simulink model "RWA_Controller"  (R2017a)
settings: Solver=VariableStepAuto  StartTime=0  StopTime=ts+60  FixedStep=0.01  RelTol=1e-3
InitFcn:
  | Init_Sim
values from neighbouring files (symbols this model uses):
  I = [0.07920140 0.00973142 0.00215335 ... (first row only)    [Init_Sim.m]
  J = Jw + Jm    (= 2.539e-05)    [Init_Sim.m]
  K = [k1  0   0   0 ... (first row only)    [Init_Sim.m]    (also in animate.m = eciunitvecs(:,3))
  Kd = 2*zeta*wn    (= 0.133333333333)    [Init_Sim.m]
  Ke = 1/(56*pi)    (= 0.00568410511042)    [Init_Sim.m]
  Kp = 2*wn^2    (= 0.00888888888889)    [Init_Sim.m]
  Kt = 5.67e-3    (= 0.00567)    [Init_Sim.m]
  phi_d = 0    [Init_Sim.m]
  phi_d0 = 0    [Init_Sim.m]
  psi_d = -90    [Init_Sim.m]
  psi_d0 = 0    [Init_Sim.m]
  r = [0.00004275; -0.00008398; -0.9099]*10^(-3)    [Init_Sim.m]    (also in csacs_nonlinear_dyn.m = [r_temp(1) r_temp(2) r_temp(3)]')
  T = [ cos(beta)            0        sin(beta) ... (first row only)    [Init_Sim.m]
  theta_d = 0    [Init_Sim.m]
  theta_d0 = 0    [Init_Sim.m]
  W = [w1   0   0   0 ... (first row only)    [Init_Sim.m]
  wn = 4/(zeta*ts)    (= 0.0666666666667)    [Init_Sim.m]
  x0 = [q_0(1); q_0(2); q_0(3); q_0(4); wb_0(1); wb_0(2); wb_0(3)]    [Init_Sim.m]
  zeta = 1    [Init_Sim.m]
settings Model: Creator=Anthony  LastModifiedBy=Anthony

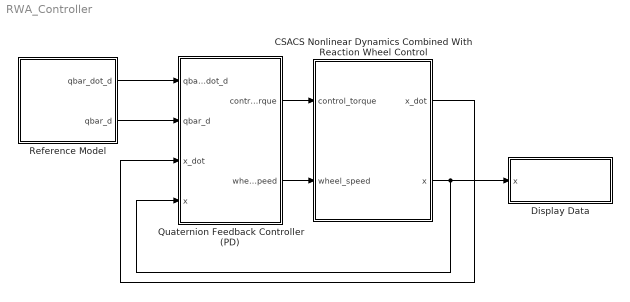
== system RWA_Controller ==
  CSACS Nonlinear Dynamics Combined With Reaction Wheel Control : Subsystem
  Display Data : Subsystem
  Quaternion Feedback Controller (PD) : Subsystem
  Reference Model : Subsystem
  wires:
  Reference Model/1(qbar_dot_d) -> Quaternion Feedback Controller (PD)/1(qbar_dot_d)
  Reference Model/2(qbar_d) -> Quaternion Feedback Controller (PD)/2(qbar_d)
  Quaternion Feedback Controller (PD)/1(control_torque) -> CSACS Nonlinear Dynamics Combined With Reaction Wheel Control/1("control_torque ")
  CSACS Nonlinear Dynamics Combined With Reaction Wheel Control/1(x_dot) -> Quaternion Feedback Controller (PD)/3(x_dot)
  CSACS Nonlinear Dynamics Combined With Reaction Wheel Control/2(x) -> Display Data/1(x), Quaternion Feedback Controller (PD)/4(x)
  Quaternion Feedback Controller (PD)/2(wheel_speed) -> CSACS Nonlinear Dynamics Combined With Reaction Wheel Control/2(wheel_speed)

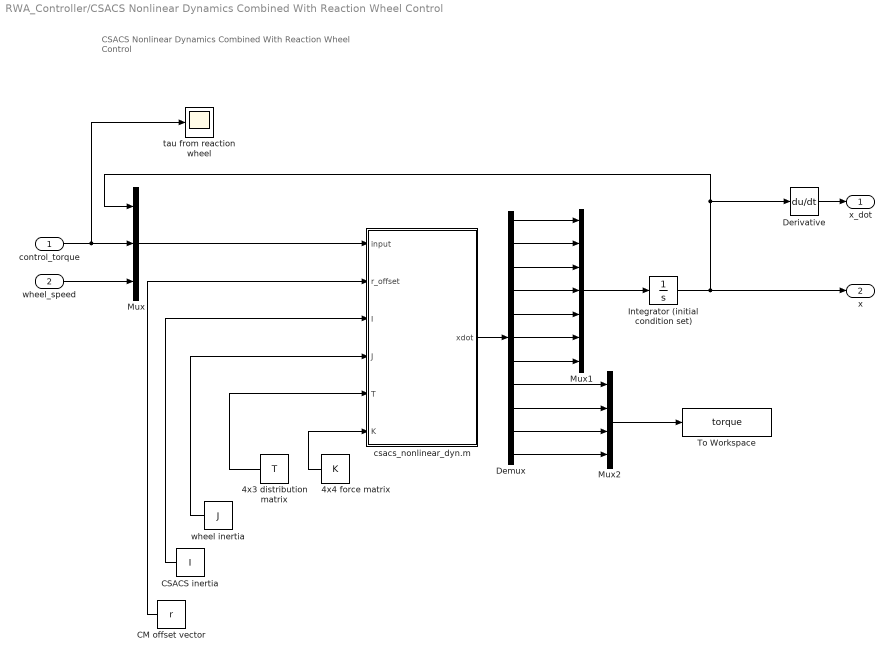
== system RWA_Controller/CSACS Nonlinear Dynamics Combined With Reaction Wheel Control ==
  note: CSACS Nonlinear Dynamics Combined
      | With Reaction Wheel Control
  "control_torque " : Inport
  wheel_speed : Inport  Port=2
  4x3 distribution matrix : Constant  Value=T  VectorParams1D=off
  4x4 force matrix : Constant  Value=K  VectorParams1D=off
  CM offset vector : Constant  Value=r  VectorParams1D=off
  CSACS inertia : Constant  Value=I  VectorParams1D=off
  Demux : Demux  Outputs=11
  Derivative : Derivative
  Integrator (initial condition set) : Integrator  InitialCondition=x0
  Mux : Mux  Inputs=3
  Mux1 : Mux  Inputs=7
  Mux2 : Mux
  To Workspace : ToWorkspace  VariableName=torque  SaveFormat=Timeseries  SampleTime=-1
  csacs_nonlinear_dyn.m : MATLAB Function  TreatAsAtomicUnit=on
  tau from reaction wheel : Scope
  wheel inertia : Constant  Value=J  VectorParams1D=off
  x_dot : Outport
  x : Outport  Port=2
  wires:
  Mux/1 -> csacs_nonlinear_dyn.m/1(input)
  "control_torque "/1 -> Mux/2, tau from reaction wheel/1
  csacs_nonlinear_dyn.m/1(xdot) -> Demux/1
  Demux/1 -> Mux1/1
  Demux/2 -> Mux1/2
  Demux/3 -> Mux1/3
  Demux/4 -> Mux1/4
  Demux/5 -> Mux1/5
  Demux/6 -> Mux1/6
  Demux/7 -> Mux1/7
  Demux/8 -> Mux2/1
  Demux/9 -> Mux2/2
  Demux/10 -> Mux2/3
  Demux/11 -> Mux2/4
  Mux1/1 -> Integrator (initial condition set)/1
  Derivative/1 -> x_dot/1
  Integrator (initial condition set)/1 -> x/1, Derivative/1, Mux/1
  Mux2/1 -> To Workspace/1
  4x4 force matrix/1 -> csacs_nonlinear_dyn.m/6(K)
  4x3 distribution matrix/1 -> csacs_nonlinear_dyn.m/5(T)
  CSACS inertia/1 -> csacs_nonlinear_dyn.m/3(I)
  CM offset vector/1 -> csacs_nonlinear_dyn.m/2(r_offset)
  wheel_speed/1 -> Mux/3
  wheel inertia/1 -> csacs_nonlinear_dyn.m/4(J)

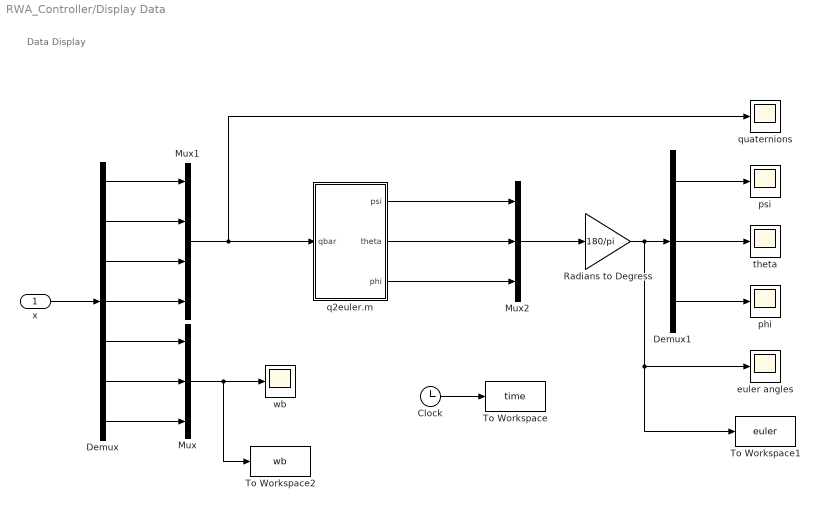
== system RWA_Controller/Display Data ==
  note: Data Display
  x : Inport
  Clock : Clock
      settings: Decimation=100
  Demux : Demux  Outputs=7
  Demux1 : Demux  Outputs=3
  Mux : Mux  Inputs=3
  Mux1 : Mux
  Mux2 : Mux  Inputs=3
  Radians to Degress : Gain  Gain=180/pi
  To Workspace : ToWorkspace  VariableName=time  SaveFormat=Timeseries  SampleTime=-1
  To Workspace1 : ToWorkspace  VariableName=euler  SaveFormat=Timeseries  SampleTime=-1
  To Workspace2 : ToWorkspace  VariableName=wb  SaveFormat=Timeseries  SampleTime=-1
  euler angles : Scope
  phi : Scope
  psi : Scope
  q2euler.m : MATLAB Function  TreatAsAtomicUnit=on
  quaternions : Scope
  theta : Scope
  wb : Scope
  wires:
  x/1 -> Demux/1
  Demux/1 -> Mux1/1
  Demux/2 -> Mux1/2
  Demux/3 -> Mux1/3
  Demux/4 -> Mux1/4
  Demux/6 -> Mux/2
  Demux/5 -> Mux/1
  Demux/7 -> Mux/3
  Demux1/1 -> psi/1
  Demux1/2 -> theta/1
  Demux1/3 -> phi/1
  Mux2/1 -> Radians to Degress/1
  Mux1/1 -> quaternions/1, q2euler.m/1(qbar)
  Clock/1 -> To Workspace/1
  Radians to Degress/1 -> euler angles/1, To Workspace1/1, Demux1/1
  Mux/1 -> To Workspace2/1, wb/1
  q2euler.m/1(psi) -> Mux2/1
  q2euler.m/2(theta) -> Mux2/2
  q2euler.m/3(phi) -> Mux2/3

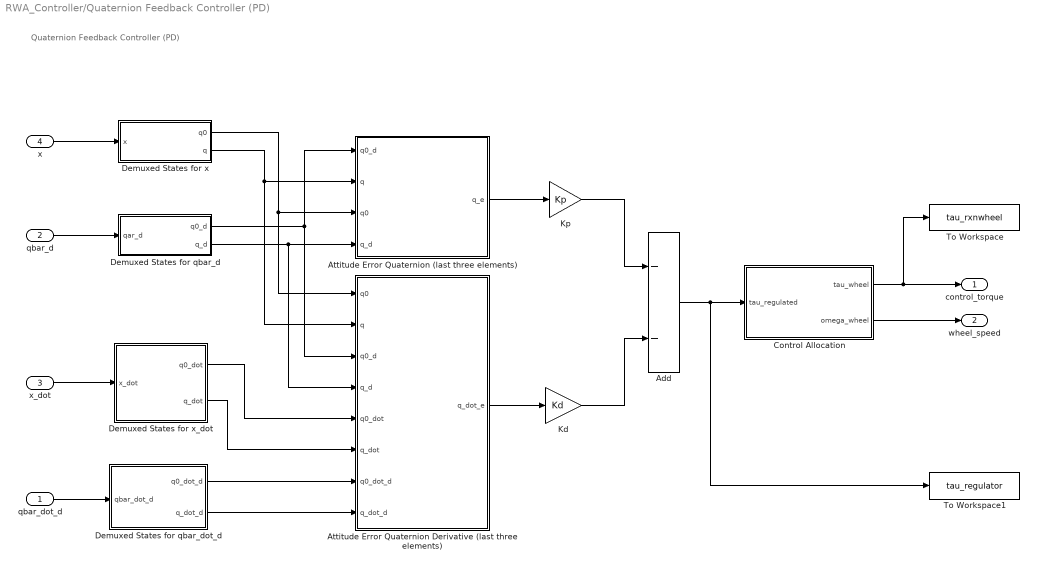
== system RWA_Controller/Quaternion Feedback Controller (PD) ==
  note: Quaternion Feedback Controller (PD)
  qbar_dot_d : Inport
  qbar_d : Inport  Port=2
  x_dot : Inport  Port=3
  x : Inport  Port=4
  Add : Sum  Inputs=--
  Attitude Error Quaternion (last three elements) : Subsystem
  Attitude Error Quaternion Derivative (last three elements) : Subsystem
  Control Allocation : Subsystem
  Demuxed States for qbar_d : Subsystem
  Demuxed States for qbar_dot_d : Subsystem
  Demuxed States for x : Subsystem
  Demuxed States for x_dot : Subsystem
  Kd : Gain  Gain=Kd
  Kp : Gain  Gain=Kp
  To Workspace : ToWorkspace  VariableName=tau_rxnwheel  SaveFormat=Timeseries  SampleTime=-1
  To Workspace1 : ToWorkspace  VariableName=tau_regulator  SaveFormat=Timeseries  SampleTime=-1
  control_torque : Outport
  wheel_speed : Outport  Port=2
  wires:
  qbar_dot_d/1 -> Demuxed States for qbar_dot_d/1(qbar_dot_d)
  qbar_d/1 -> Demuxed States for qbar_d/1(qar_d)
  x_dot/1 -> Demuxed States for x_dot/1(x_dot)
  x/1 -> Demuxed States for x/1(x)
  Demuxed States for x/1(q0) -> Attitude Error Quaternion Derivative (last three elements)/1(q0), Attitude Error Quaternion (last three elements)/3(q0)
  Demuxed States for x/2(q) -> Attitude Error Quaternion Derivative (last three elements)/2(q), Attitude Error Quaternion (last three elements)/2(q)
  Demuxed States for qbar_d/1(q0_d) -> Attitude Error Quaternion Derivative (last three elements)/3(q0_d), Attitude Error Quaternion (last three elements)/1(q0_d)
  Demuxed States for qbar_d/2(q_d) -> Attitude Error Quaternion Derivative (last three elements)/4(q_d), Attitude Error Quaternion (last three elements)/4(q_d)
  Demuxed States for qbar_dot_d/2(q_dot_d) -> Attitude Error Quaternion Derivative (last three elements)/8(q_dot_d)
  Demuxed States for qbar_dot_d/1(q0_dot_d) -> Attitude Error Quaternion Derivative (last three elements)/7(q0_dot_d)
  Demuxed States for x_dot/1(q0_dot) -> Attitude Error Quaternion Derivative (last three elements)/5(q0_dot)
  Demuxed States for x_dot/2(q_dot) -> Attitude Error Quaternion Derivative (last three elements)/6(q_dot)
  Attitude Error Quaternion Derivative (last three elements)/1(q_dot_e) -> Kd/1
  Attitude Error Quaternion (last three elements)/1(q_e) -> Kp/1
  Kp/1 -> Add/1
  Kd/1 -> Add/2
  Control Allocation/1(tau_wheel) -> control_torque/1, To Workspace/1
  Add/1 -> To Workspace1/1, Control Allocation/1(tau_regulated)
  Control Allocation/2(omega_wheel) -> wheel_speed/1

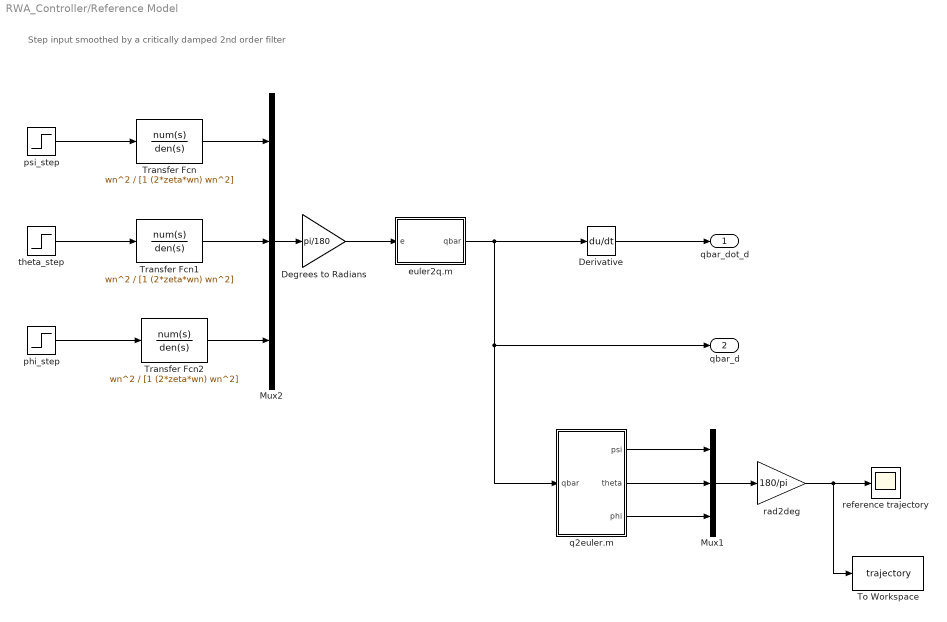
== system RWA_Controller/Reference Model ==
  note: Step input smoothed by a critically damped 2nd order filter
  Degrees to Radians : Gain  Gain=pi/180
  Derivative : Derivative
  Mux1 : Mux  Inputs=3
  Mux2 : Mux  Inputs=3
  To Workspace : ToWorkspace  VariableName=trajectory  SaveFormat=Timeseries  SampleTime=-1
  Transfer Fcn : TransferFcn  Numerator=wn^2  Denominator=[1 (2*zeta*wn) wn^2]
  Transfer Fcn1 : TransferFcn  Numerator=wn^2  Denominator=[1 (2*zeta*wn) wn^2]
  Transfer Fcn2 : TransferFcn  Numerator=wn^2  Denominator=[1 (2*zeta*wn) wn^2]
  euler2q.m : MATLAB Function  TreatAsAtomicUnit=on
  phi_step : Step  Before=phi_d0  After=phi_d  SampleTime=0
  "psi_step " : Step  Before=psi_d0  After=psi_d  SampleTime=0
  q2euler.m : MATLAB Function  TreatAsAtomicUnit=on
  rad2deg : Gain  Gain=180/pi
  reference trajectory : Scope
  theta_step : Step  Before=theta_d0  After=theta_d  SampleTime=0
  qbar_dot_d : Outport
  qbar_d : Outport  Port=2
  wires:
  theta_step/1 -> Transfer Fcn1/1
  Transfer Fcn2/1 -> Mux2/3
  Transfer Fcn1/1 -> Mux2/2
  phi_step/1 -> Transfer Fcn2/1
  "psi_step "/1 -> Transfer Fcn/1
  euler2q.m/1(qbar) -> qbar_d/1, q2euler.m/1(qbar), Derivative/1
  q2euler.m/2(theta) -> Mux1/2
  Degrees to Radians/1 -> euler2q.m/1(e)
  rad2deg/1 -> To Workspace/1, reference trajectory/1
  q2euler.m/1(psi) -> Mux1/1
  q2euler.m/3(phi) -> Mux1/3
  Derivative/1 -> qbar_dot_d/1
  Mux1/1 -> rad2deg/1
  Mux2/1 -> Degrees to Radians/1
  Transfer Fcn/1 -> Mux2/1

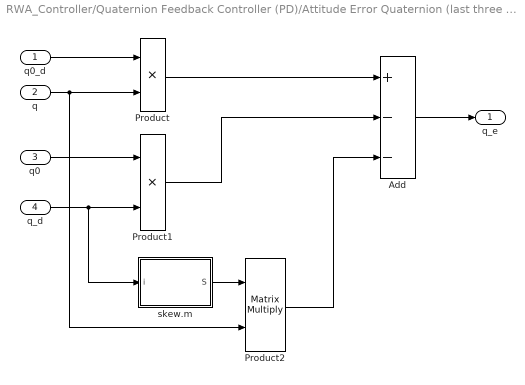
== system RWA_Controller/Quaternion Feedback Controller (PD)/Attitude Error Quaternion (last three elements) ==
  q0_d : Inport
  q : Inport  Port=2
  q0 : Inport  Port=3
  q_d : Inport  Port=4
  Add : Sum  Inputs=+--
  Product : Product
  Product1 : Product
  Product2 : Product  Multiplication=Matrix(*)
  skew.m : MATLAB Function  TreatAsAtomicUnit=on
  q_e : Outport
  wires:
  skew.m/1(S) -> Product2/1
  q0_d/1 -> Product/1
  q0/1 -> Product1/1
  q_d/1 -> skew.m/1(i), Product1/2
  q/1 -> Product2/2, Product/2
  Product/1 -> Add/1
  Product1/1 -> Add/2
  Add/1 -> q_e/1
  Product2/1 -> Add/3

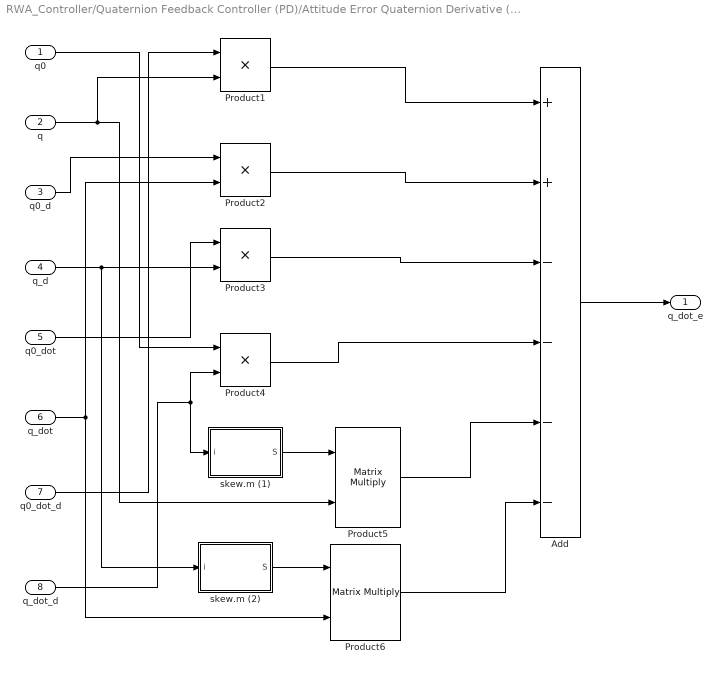
== system RWA_Controller/Quaternion Feedback Controller (PD)/Attitude Error Quaternion Derivative (last three elements) ==
  q0 : Inport
  q : Inport  Port=2
  q0_d : Inport  Port=3
  q_d : Inport  Port=4
  q0_dot : Inport  Port=5
  q_dot : Inport  Port=6
  q0_dot_d : Inport  Port=7
  q_dot_d : Inport  Port=8
  Add : Sum  Inputs=++----
  Product{1..4} (4 alike) : Product
  Product5 : Product  Multiplication=Matrix(*)
  Product6 : Product  Multiplication=Matrix(*)
  skew.m (1) : MATLAB Function  TreatAsAtomicUnit=on
  skew.m (2) : MATLAB Function  TreatAsAtomicUnit=on
  q_dot_e : Outport
  wires:
  Add/1 -> q_dot_e/1
  q0/1 -> Product4/1
  q_dot_d/1 -> skew.m (1)/1(i), Product4/2
  q_d/1 -> skew.m (2)/1(i), Product3/2
  q0_dot/1 -> Product3/1
  q0_dot_d/1 -> Product1/1
  skew.m (2)/1(S) -> Product6/1
  q_dot/1 -> Product6/2, Product2/2
  skew.m (1)/1(S) -> Product5/1
  q/1 -> Product5/2, Product1/2
  q0_d/1 -> Product2/1
  Product1/1 -> Add/1
  Product2/1 -> Add/2
  Product3/1 -> Add/3
  Product4/1 -> Add/4
  Product5/1 -> Add/5
  Product6/1 -> Add/6

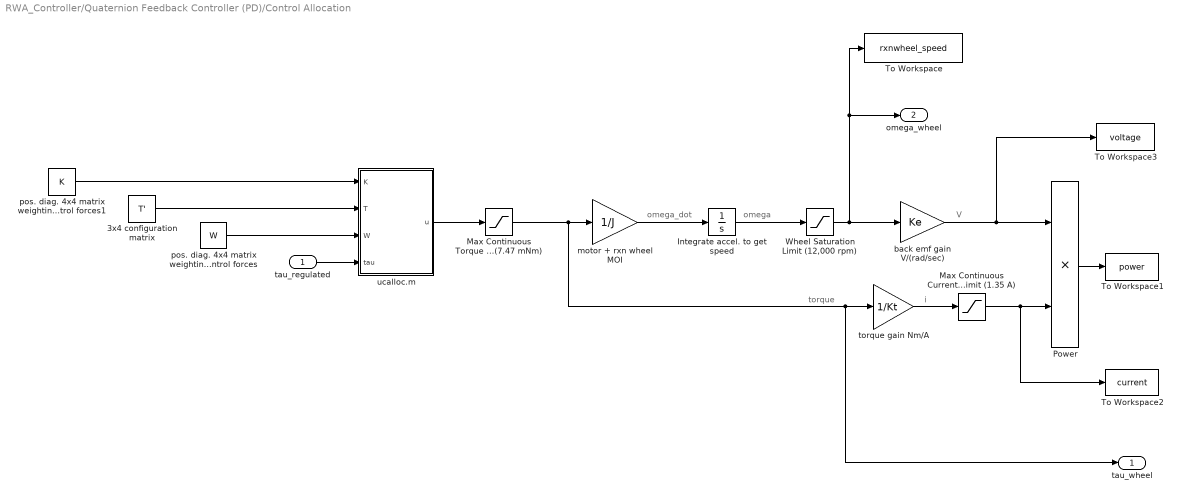
== system RWA_Controller/Quaternion Feedback Controller (PD)/Control Allocation ==
  note: torque
  note: omega
  note: omega_dot
  note: i
  note: V
  tau_regulated : Inport
  3x4 configuration matrix : Constant  Value=T'  VectorParams1D=off
  Integrate accel. to get speed : Integrator
  Max Continuous Current Limit (1.35 A) : Saturate  UpperLimit=12e3*(pi/30)  LowerLimit=-12e3*(pi/30)
  Max Continuous Torque Limit (7.47 mNm) : Saturate  UpperLimit=7.47e-3  LowerLimit=-7.47e-3
  Power : Product
  To Workspace : ToWorkspace  VariableName=rxnwheel_speed  SaveFormat=Timeseries  SampleTime=-1
  To Workspace1 : ToWorkspace  VariableName=power  SaveFormat=Timeseries  SampleTime=-1
  To Workspace2 : ToWorkspace  VariableName=current  SaveFormat=Timeseries  SampleTime=-1
  To Workspace3 : ToWorkspace  VariableName=voltage  SaveFormat=Timeseries  SampleTime=-1
  Wheel Saturation Limit (12,000 rpm) : Saturate  UpperLimit=12e3*(pi/30)  LowerLimit=-12e3*(pi/30)
  back emf gain V/(rad/sec) : Gain  Gain=Ke
  motor + rxn wheel MOI : Gain  Gain=1/J
  pos. diag. 4x4 matrix weighting the control forces : Constant  Value=W  VectorParams1D=off
  pos. diag. 4x4 matrix weighting the control forces1 : Constant  Value=K  VectorParams1D=off
  torque gain Nm/A : Gain  Gain=1/Kt
  ucalloc.m : MATLAB Function  TreatAsAtomicUnit=on
  tau_wheel : Outport
  omega_wheel : Outport  Port=2
  wires:
  tau_regulated/1 -> ucalloc.m/4(tau)
  ucalloc.m/1(u) -> Max Continuous Torque Limit (7.47 mNm)/1
  pos. diag. 4x4 matrix weighting the control forces1/1 -> ucalloc.m/1(K)
  3x4 configuration matrix/1 -> ucalloc.m/2(T)
  pos. diag. 4x4 matrix weighting the control forces/1 -> ucalloc.m/3(W)
  motor + rxn wheel MOI/1 -> Integrate accel. to get speed/1
  Integrate accel. to get speed/1 -> Wheel Saturation Limit (12,000 rpm)/1
  back emf gain V/(rad/sec)/1 -> To Workspace3/1, Power/1
  Power/1 -> To Workspace1/1
  Wheel Saturation Limit (12,000 rpm)/1 -> back emf gain V/(rad/sec)/1, omega_wheel/1, To Workspace/1
  Max Continuous Torque Limit (7.47 mNm)/1 -> tau_wheel/1, torque gain Nm/A/1, motor + rxn wheel MOI/1
  torque gain Nm/A/1 -> Max Continuous Current Limit (1.35 A)/1
  Max Continuous Current Limit (1.35 A)/1 -> To Workspace2/1, Power/2

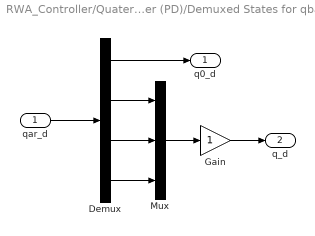
== system RWA_Controller/Quaternion Feedback Controller (PD)/Demuxed States for qbar_d ==
  qar_d : Inport
  Demux : Demux
  Gain : Gain
  Mux : Mux  Inputs=3
  q0_d : Outport
  q_d : Outport  Port=2
  wires:
  qar_d/1 -> Demux/1
  Demux/1 -> q0_d/1
  Demux/2 -> Mux/1
  Demux/3 -> Mux/2
  Demux/4 -> Mux/3
  Mux/1 -> Gain/1
  Gain/1 -> q_d/1

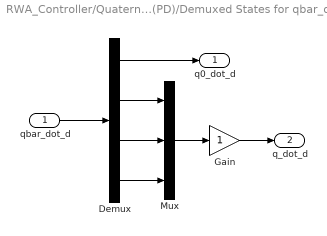
== system RWA_Controller/Quaternion Feedback Controller (PD)/Demuxed States for qbar_dot_d ==
  qbar_dot_d : Inport
  Demux : Demux
  Gain : Gain
  Mux : Mux  Inputs=3
  q0_dot_d : Outport
  q_dot_d : Outport  Port=2
  wires:
  qbar_dot_d/1 -> Demux/1
  Demux/1 -> q0_dot_d/1
  Demux/2 -> Mux/1
  Demux/3 -> Mux/2
  Demux/4 -> Mux/3
  Mux/1 -> Gain/1
  Gain/1 -> q_dot_d/1

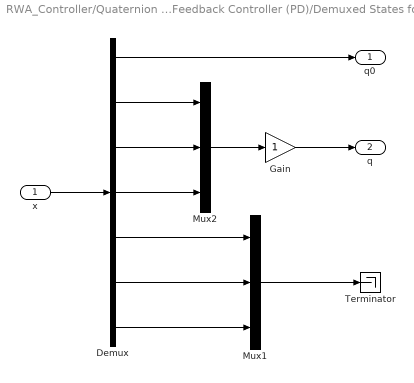
== system RWA_Controller/Quaternion Feedback Controller (PD)/Demuxed States for x ==
  x : Inport
  Demux : Demux  Outputs=7
  Gain : Gain
  Mux1 : Mux  Inputs=3
  Mux2 : Mux  Inputs=3
  Terminator : Terminator
  q0 : Outport
  q : Outport  Port=2
  wires:
  x/1 -> Demux/1
  Demux/1 -> q0/1
  Demux/6 -> Mux1/2
  Demux/7 -> Mux1/3
  Demux/5 -> Mux1/1
  Demux/2 -> Mux2/1
  Demux/3 -> Mux2/2
  Demux/4 -> Mux2/3
  Mux2/1 -> Gain/1
  Mux1/1 -> Terminator/1
  Gain/1 -> q/1

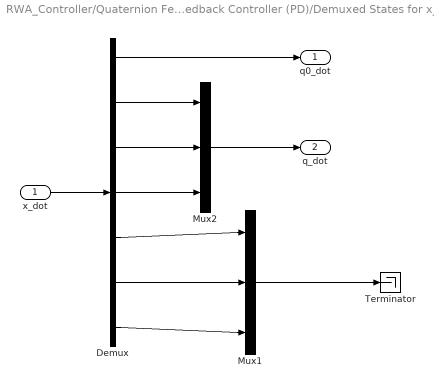
== system RWA_Controller/Quaternion Feedback Controller (PD)/Demuxed States for x_dot ==
  x_dot : Inport
  Demux : Demux  Outputs=7
  Mux1 : Mux  Inputs=3
  Mux2 : Mux  Inputs=3
  Terminator : Terminator
  q0_dot : Outport
  q_dot : Outport  Port=2
  wires:
  x_dot/1 -> Demux/1
  Demux/1 -> q0_dot/1
  Demux/6 -> Mux1/2
  Demux/7 -> Mux1/3
  Demux/5 -> Mux1/1
  Demux/2 -> Mux2/1
  Demux/3 -> Mux2/2
  Demux/4 -> Mux2/3
  Mux2/1 -> q_dot/1
  Mux1/1 -> Terminator/1

== matlab function RWA_Controller/Quaternion Feedback Controller (PD)/Attitude Error Quaternion Derivative (last three elements)/skew.m (1) ==
  data: i input; S output
%*********************************************************************
% skew.m
% Function that takes skew symmetric matrix of input
% (i denotes the input matrix)
%*********************************************************************
function S = skew(i)

S =[  0  -i(3)   i(2);
    i(3)    0   -i(1)
   -i(2)  i(1)     0];

end

== matlab function RWA_Controller/Reference Model/euler2q.m ==
  data: e input; qbar output
%*********************************************************************
% euler2q.m
% Transforms Euler angles to quaternion parameters via a 3-2-1 sequence. 
% Meaning psi is the first rotation, theta is the second rotation, and phi
% is the third rotation 
%*********************************************************************
function qbar = euler2q(e)

k1   = 0.5*e(1);  % psi (yaw)
k2   = 0.5*e(2);  % theta (pitch)
k3   = 0.5*e(3);  % phi (roll)

cy   = cos(k1);
sy   = sin(k1);
cp   = cos(k2);
sp   = sin(k2);
cr   = cos(k3);
sr   = sin(k3);

q0   = cy * cr * cp + sy * sr * sp;
q1   = cy * sr * cp - sy * cr * sp;
q2   = cy * cr * sp + sy * sr * cp;
q3   = sy * cr * cp - cy * sr * sp;

qbar = [q0; q1; q2; q3];

end

== matlab function RWA_Controller/Quaternion Feedback Controller (PD)/Attitude Error Quaternion Derivative (last three elements)/skew.m (2) ==
  data: i input; S output
%*********************************************************************
% skew.m
% Function that takes skew symmetric matrix of input
% (i denotes the input matrix)
%*********************************************************************
function S = skew(i)

S =[  0  -i(3)   i(2);
    i(3)    0   -i(1)
   -i(2)  i(1)     0];

end

== matlab function RWA_Controller/CSACS Nonlinear Dynamics Combined With Reaction Wheel Control/csacs_nonlinear_dyn.m ==
  data: input input; xdot output; r_offset input; I input; J input; T input; K input
%*********************************************************************
% csacs_nonlinear_dyn.m
% A file to calculate the nonlinear dynamic equations of the CSACS, 
% coupled with the RWA
%*********************************************************************
function xdot = csacs_nonlinear_dyn(input,r_offset,I,J,T,K)

%*********************************************************************
% Reassign Input Variables
%*********************************************************************
% Attitude quaternions
qbar_temp = input(1:4);
qbar      = [qbar_temp(1) qbar_temp(2) qbar_temp(3) qbar_temp(4)]';

% Body rates
w_temp    = input(5:7);
wb        = [w_temp(1) w_temp(2) w_temp(3)]';

% Control torques
u_temp    = input(8:11);
u         = [u_temp(1) u_temp(2) u_temp(3) u_temp(4)]';

% Wheel speeds
ww_temp   = input(12:15);
ww        = [ww_temp(1) ww_temp(2) ww_temp(3) ww_temp(4)]';

% Normalizing the quaternions - necessary for numerical accuracy
qbar      = qbar/(qbar'*qbar);
q0        = qbar(1);
q         = qbar(2:4);

%*********************************************************************
% Reaction Wheel Torque and Angular Momentum Redistribution
%*********************************************************************
Tc = T'*K*u;
hw = J*(T'*K*ww);

%*********************************************************************
% Gravitational Torque Contribution
%*********************************************************************
% CM offset vector
r_temp = r_offset(1:3);
r      = [r_temp(1) r_temp(2) r_temp(3)]';

m      = 7.75345629;        % total mass of the CSACS [kg]
g      = 9.81;              % acceleration due to gravity [m/s^2]

% Gravitational torque from when the CSACS is not centered on the CR (NOTE:
% both methods produce identical results, i.e., using euler angles vs.
% using quaternions -- comment out one method, and use the other)

% using euler angles:
% [~,theta,phi] = q2euler(qbar);
% Tg = m*g*[-r(2)*cos(theta)*cos(phi) + r(3)*sin(phi)*cos(theta);
%           r(3)*sin(theta)           + r(1)*cos(phi)*cos(theta);
%           -r(1)*sin(phi)*cos(theta) -          r(2)*sin(theta)];

% using quaternions:
R = Rquat(qbar);
Tg = -m*g*skew([r(1); r(2); r(3)])*R*[0; 0; 1];
      
%*********************************************************************
% Aerodynamic Torque Contribution
%*********************************************************************
% aerodynamic damping coeff (neglect for control model)
b     = [0; 0; 0]; 
Taero = -[b(1)*wb(1)^2; b(2)*wb(2)^2; b(3)*wb(3)^2];

%*********************************************************************
% Output Time Derivatives of X (from full, nonlinear equations of motion)
%*********************************************************************
% Kinematics
q0_dot = -(1/2)*q'*wb;
q_dot  = (1/2)*(q0*eye(3) + skew(q))*wb;

% Attitude dynamics of the CSACS
wb_dot = inv(I)*(Tc + Tg + Taero - skew(wb)*(I*wb + hw));

xdot = [q0_dot; q_dot; wb_dot; u];

== matlab function RWA_Controller/Display Data/q2euler.m ==
  data: qbar input; psi output; theta output; phi output
%*********************************************************************
% q2euler.m
% Computes the Euler angles from the unit quaternions qbar = [q0 q1 q2 q3]'
% via a 3-2-1 sequence, meaning psi is the first rotation, theta is the 
% second rotation, and phi is the third rotation 
%*********************************************************************
function [psi,theta,phi] = q2euler(qbar)

q0  = qbar(1);
q1  = qbar(2);
q2  = qbar(3);
q3  = qbar(4);
 
R = Rquat(qbar);
if abs(R(3,1)) > 1.0
    error('solution is singular for theta = +- 90 degrees'); 
end

% Expanded terms (same as below)
% psi   = atan2(2*(q0*q3 + q1*q2), (q0^2 + q1^2 - q2^2 - q3^2));
% theta = asin(2*(q0*q2 - q3*q1));
% phi   = atan2(2*(q0*q1 + q2*q3), (q0^2 - q1^2 - q2^2 + q3^2));

psi   = atan2(R(1,2),R(1,1));
theta = asin(-R(1,3));
phi   = atan2(R(2,3),R(3,3));

== matlab function RWA_Controller/Quaternion Feedback Controller (PD)/Attitude Error Quaternion (last three elements)/skew.m ==
  data: i input; S output
%*********************************************************************
% skew.m
% Function that takes skew symmetric matrix of input
% (i denotes the input matrix)
%*********************************************************************
function S = skew(i)

S =[  0  -i(3)   i(2);
    i(3)    0   -i(1)
   -i(2)  i(1)     0];

end

== matlab function RWA_Controller/Quaternion Feedback Controller (PD)/Control Allocation/ucalloc.m ==
  data: K input; T input; W input; u output; tau input
%*********************************************************************
% ucalloc.m
% Unconstrained control allocation function. The generalized force vector 
% tau = T*K*u (dim n) is distributed to the input vector u (dim r), 
% where r>=n by minimizing the force f=K*u.
%
% An unconstrained solution u = inv(K)*inv(W)*T'*inv(T*inv(W)*T')
% exists if T*T' is non-singular. 
%
%   - K is a diagonal rxr matrix of force coeffisients 
%   - T is a nxr constant configuration matrix. 
%   - W is a rxr positive diagonal matrix weighting (prizing) the 
%     different control forces f = K*u.
%
% Adapted from the Marine Guidance, Navigation and Control Toolbox
%
% Author:    Thor I. Fossen
% Date:      3rd November 2001
% Revisions: 25th September 2002 - function name changed from alloc.m to ucalloc.m
%
% Copyright (C) 2008 Thor I. Fossen and Tristan Perez
%*********************************************************************
function u = ucalloc(K,T,W,tau)

tau = [tau(1) tau(2) tau(3)]';

if det(T*T') == 0 
    error('T*T''is singular'); 
elseif det(W)==0
    error('W must be positive'); 
else
    Winv = inv(W);
    u    = inv(K)*Winv*T'*inv(T*Winv*T')*tau;
end

== matlab function RWA_Controller/Reference Model/q2euler.m ==
  data: qbar input; psi output; theta output; phi output
%*********************************************************************
% q2euler.m
% Computes the Euler angles from the unit quaternions qbar = [q0 q1 q2 q3]'
% via a 3-2-1 sequence, meaning psi is the first rotation, theta is the 
% second rotation, and phi is the third rotation 
%*********************************************************************
function [psi,theta,phi] = q2euler(qbar)

q0  = qbar(1);
q1  = qbar(2);
q2  = qbar(3);
q3  = qbar(4);
 
R = Rquat(qbar);
if abs(R(3,1)) > 1.0
    error('solution is singular for theta = +- 90 degrees'); 
end

% Expanded terms (same as below)
% psi   = atan2(2*(q0*q3 + q1*q2), (q0^2 + q1^2 - q2^2 - q3^2));
% theta = asin(2*(q0*q2 - q3*q1));
% phi   = atan2(2*(q0*q1 + q2*q3), (q0^2 - q1^2 - q2^2 + q3^2));

psi   = atan2(R(1,2),R(1,1));
theta = asin(-R(1,3));
phi   = atan2(R(2,3),R(3,3));
